simulink library "Atmospheric_lib"  (R2020a)
settings: Solver=VariableStepAuto  StartTime=0.0  StopTime=10.0  RelTol=1e-3
settings Model: Creator=muril  LastModifiedBy=muril

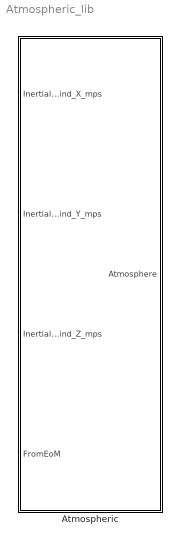
== system Atmospheric_lib ==
  Atmospheric : Subsystem

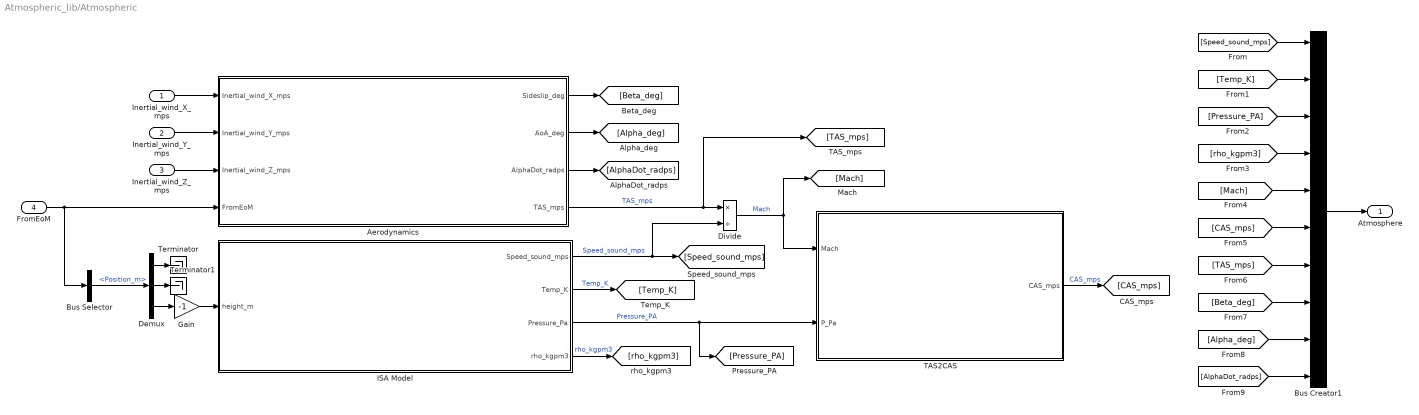
== system Atmospheric_lib/Atmospheric ==
  Inertial_wind_X_mps : Inport
  Inertial_wind_Y_mps : Inport  Port=2
  Inertial_wind_Z_mps : Inport  Port=3
  FromEoM : Inport  Port=4
  Aerodynamics : Subsystem
  Bus Creator1 : BusCreator  Inputs=10
  Bus Selector : BusSelector  OutputSignals=Position_m
  Demux : Demux  Outputs=3
  Divide : Product  Inputs=*/
  Gain : Gain  Gain=-1
  ISA Model : Subsystem
  TAS2CAS : Subsystem
  Terminator : Terminator
  Terminator1 : Terminator
  Atmosphere : Outport
  wires:
  Gain/1 -> ISA Model/1(height_m)
  Bus Selector/1 -> Demux/1  "<Position_m>"
  Demux/2 -> Terminator1/1
  Demux/1 -> Terminator/1
  Demux/3 -> Gain/1
  FromEoM/1 -> Bus Selector/1, Aerodynamics/4(FromEoM)
  Aerodynamics/4(TAS_mps) -> [TAS_mps], Divide/1  "TAS_mps"
  [Speed_sound_mps] -> Bus Creator1/1
  [TAS_mps] -> Bus Creator1/7
  ISA Model/3(Pressure_Pa) -> TAS2CAS/2(P_Pa), [Pressure_PA]  "Pressure_PA"
  ISA Model/4(rho_kgpm3) -> [rho_kgpm3]  "rho_kgpm3"
  ISA Model/1(Speed_sound_mps) -> [Speed_sound_mps], Divide/2  "Speed_sound_mps"
  Aerodynamics/3(AlphaDot_radps) -> [AlphaDot_radps]
  [Pressure_PA] -> Bus Creator1/3
  Divide/1 -> [Mach], TAS2CAS/1(Mach)  "Mach"
  [Alpha_deg] -> Bus Creator1/9
  Inertial_wind_Z_mps/1 -> Aerodynamics/3(Inertial_wind_Z_mps)
  Aerodynamics/1(Sideslip_deg) -> [Beta_deg]
  ISA Model/2(Temp_K) -> [Temp_K]  "Temp_K"
  Aerodynamics/2(AoA_deg) -> [Alpha_deg]
  TAS2CAS/1(CAS_mps) -> [CAS_mps]  "CAS_mps"
  [CAS_mps] -> Bus Creator1/6
  [rho_kgpm3] -> Bus Creator1/4
  Inertial_wind_Y_mps/1 -> Aerodynamics/2(Inertial_wind_Y_mps)
  Inertial_wind_X_mps/1 -> Aerodynamics/1(Inertial_wind_X_mps)
  [AlphaDot_radps] -> Bus Creator1/10
  Bus Creator1/1 -> Atmosphere/1
  [Beta_deg] -> Bus Creator1/8
  [Temp_K] -> Bus Creator1/2
  [Mach] -> Bus Creator1/5

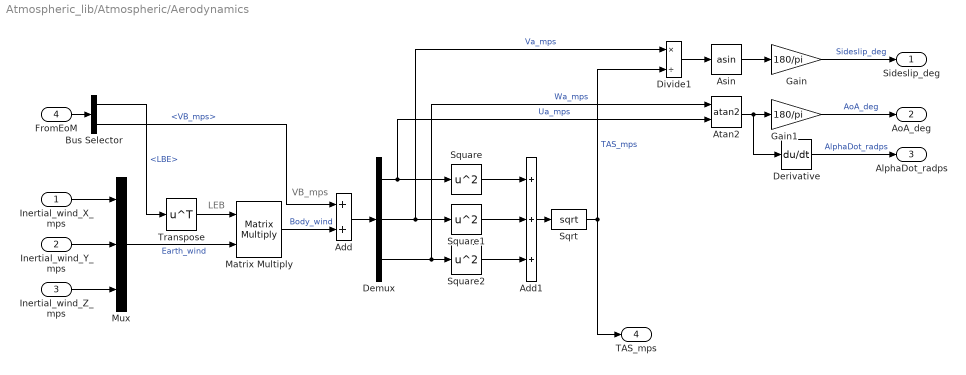
== system Atmospheric_lib/Atmospheric/Aerodynamics ==
  note: LEB
  note: VB_mps
  Inertial_wind_X_mps : Inport
  Inertial_wind_Y_mps : Inport  Port=2
  Inertial_wind_Z_mps : Inport  Port=3
  FromEoM : Inport  Port=4
  Add : Sum
  Add1 : Sum  Inputs=+++
  Asin : Trigonometry  Operator=asin
  Atan2 : Trigonometry  Operator=atan2
  Bus Selector : BusSelector  OutputSignals=LBE,VB_mps
  Demux : Demux  Outputs=3
  Derivative : Derivative
  Divide1 : Product  Inputs=*/
  Gain : Gain  Gain=180/pi
  Gain1 : Gain  Gain=180/pi
  Matrix Multiply : Product  Multiplication=Matrix(*)
  Mux : Mux  Inputs=3
  Sqrt : Sqrt  SaturateOnIntegerOverflow=on
  Square : Math  Operator=square  SaturateOnIntegerOverflow=on
  Square1 : Math  Operator=square  SaturateOnIntegerOverflow=on
  Square2 : Math  Operator=square  SaturateOnIntegerOverflow=on
  Transpose : Math  Operator=transpose  SaturateOnIntegerOverflow=on
  Sideslip_deg : Outport
  AoA_deg : Outport  Port=2
  AlphaDot_radps : Outport  Port=3
  TAS_mps : Outport  Port=4
  wires:
  Derivative/1 -> AlphaDot_radps/1  "AlphaDot_radps"
  Gain/1 -> Sideslip_deg/1  "Sideslip_deg"
  Divide1/1 -> Asin/1
  Inertial_wind_Y_mps/1 -> Mux/2
  Transpose/1 -> Matrix Multiply/1
  Bus Selector/1 -> Transpose/1  "<LBE>"
  Sqrt/1 -> TAS_mps/1, Divide1/2  "TAS_mps"
  Demux/2 -> Square1/1, Divide1/1  "Va_mps"
  Inertial_wind_Z_mps/1 -> Mux/3
  Demux/1 -> Atan2/2, Square/1  "Ua_mps"
  Square/1 -> Add1/1
  Demux/3 -> Square2/1, Atan2/1  "Wa_mps"
  Add1/1 -> Sqrt/1
  Asin/1 -> Gain/1
  Square2/1 -> Add1/3
  Add/1 -> Demux/1
  FromEoM/1 -> Bus Selector/1
  Square1/1 -> Add1/2
  Inertial_wind_X_mps/1 -> Mux/1
  Mux/1 -> Matrix Multiply/2  "Earth_wind"
  Matrix Multiply/1 -> Add/2  "Body_wind"
  Bus Selector/2 -> Add/1  "<VB_mps>"
  Atan2/1 -> Gain1/1, Derivative/1
  Gain1/1 -> AoA_deg/1  "AoA_deg"

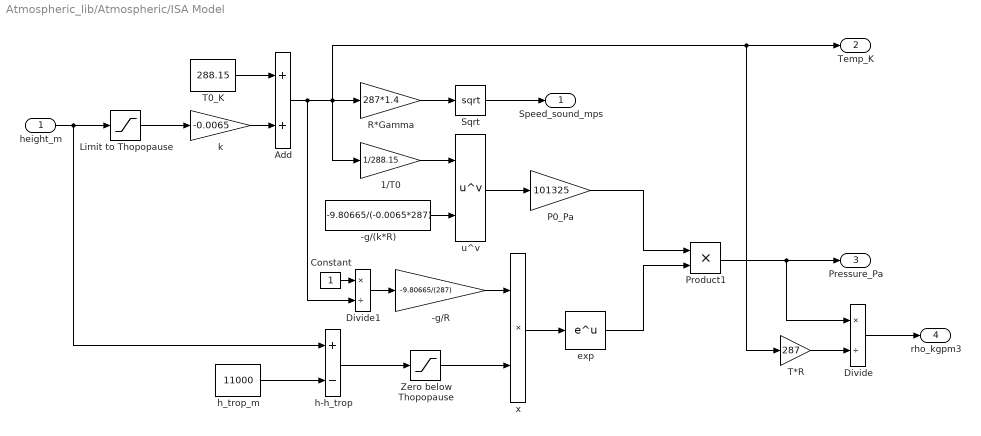
== system Atmospheric_lib/Atmospheric/ISA Model ==
  height_m : Inport
  -g/(k*R) : Constant  Value=-9.80665/(-0.0065*287)
  -g/R : Gain  Gain=-9.80665/(287)
  1/T0 : Gain  Gain=1/288.15
  Add : Sum
  Constant : Constant
  Divide : Product  Inputs=*/
  Divide1 : Product  Inputs=*/
  Limit to Thopopause : Saturate  UpperLimit=11000  LowerLimit=0
  P0_Pa : Gain  Gain=101325
  Product1 : Product
  R*Gamma : Gain  Gain=287*1.4
  Sqrt : Sqrt  SaturateOnIntegerOverflow=on
  T*R : Gain  Gain=287
  T0_K : Constant  Value=288.15
  Zero below Thopopause : Saturate  UpperLimit=inf  LowerLimit=0
  exp : Math  SaturateOnIntegerOverflow=on
  h-h_trop : Sum  Inputs=+-
  h_trop_m : Constant  Value=11000
  k : Gain  Gain=-0.0065
  u^v : Math  Operator=pow  SaturateOnIntegerOverflow=on
  x : Product
  Speed_sound_mps : Outport
  Temp_K : Outport  Port=2
  Pressure_Pa : Outport  Port=3
  rho_kgpm3 : Outport  Port=4
  wires:
  k/1 -> Add/2
  height_m/1 -> Limit to Thopopause/1, h-h_trop/1
  R*Gamma/1 -> Sqrt/1
  Add/1 -> Divide1/2, Temp_K/1, T*R/1, 1/T0/1, R*Gamma/1
  Sqrt/1 -> Speed_sound_mps/1
  T0_K/1 -> Add/1
  Limit to Thopopause/1 -> k/1
  -g/R/1 -> x/1
  -g/(k*R)/1 -> u^v/2
  Zero below Thopopause/1 -> x/2
  Divide/1 -> rho_kgpm3/1
  T*R/1 -> Divide/2
  Divide1/1 -> -g/R/1
  Product1/1 -> Pressure_Pa/1, Divide/1
  1/T0/1 -> u^v/1
  u^v/1 -> P0_Pa/1
  P0_Pa/1 -> Product1/1
  exp/1 -> Product1/2
  h-h_trop/1 -> Zero below Thopopause/1
  x/1 -> exp/1
  h_trop_m/1 -> h-h_trop/2
  Constant/1 -> Divide1/1

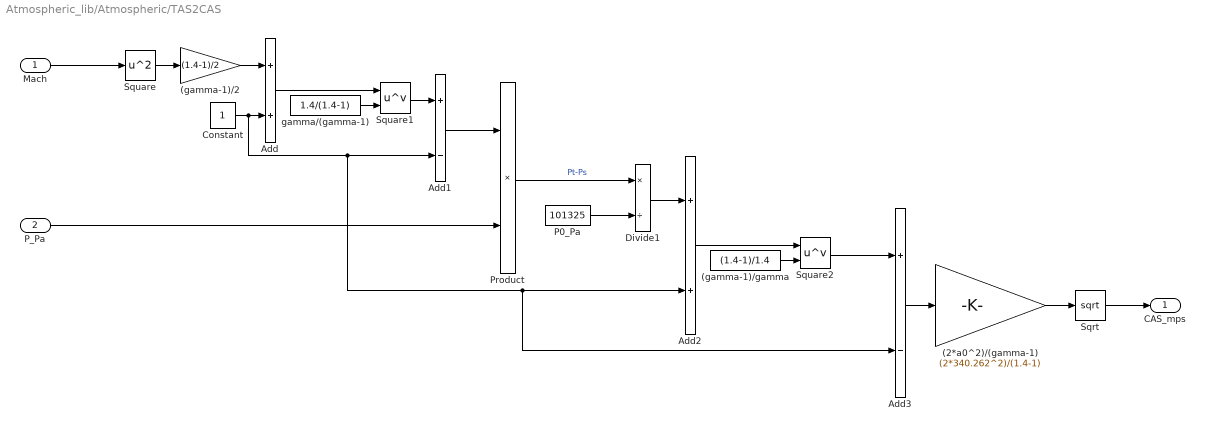
== system Atmospheric_lib/Atmospheric/TAS2CAS ==
  Mach : Inport
  P_Pa : Inport  Port=2
  (2*a0^2)/(gamma-1) : Gain  Gain=(2*340.262^2)/(1.4-1)
  (gamma-1)/2 : Gain  Gain=(1.4-1)/2
  (gamma-1)/gamma : Constant  Value=(1.4-1)/1.4
  Add : Sum
  Add1 : Sum  Inputs=+-
  Add2 : Sum
  Add3 : Sum  Inputs=+-
  Constant : Constant
  Divide1 : Product  Inputs=*/
  P0_Pa : Constant  Value=101325
  Product : Product
  Sqrt : Sqrt  SaturateOnIntegerOverflow=on
  Square : Math  Operator=square  SaturateOnIntegerOverflow=on
  Square1 : Math  Operator=pow  SaturateOnIntegerOverflow=on
  Square2 : Math  Operator=pow  SaturateOnIntegerOverflow=on
  gamma/(gamma-1) : Constant  Value=1.4/(1.4-1)
  CAS_mps : Outport
  wires:
  Constant/1 -> Add3/2, Add2/2, Add1/2, Add/2
  gamma/(gamma-1)/1 -> Square1/2
  Add3/1 -> (2*a0^2)/(gamma-1)/1
  P0_Pa/1 -> Divide1/2
  (gamma-1)/2/1 -> Add/1
  Square1/1 -> Add1/1
  Add/1 -> Square1/1
  Square/1 -> (gamma-1)/2/1
  Sqrt/1 -> CAS_mps/1
  (2*a0^2)/(gamma-1)/1 -> Sqrt/1
  (gamma-1)/gamma/1 -> Square2/2
  Add1/1 -> Product/1
  Add2/1 -> Square2/1
  Product/1 -> Divide1/1  "Pt-Ps"
  Divide1/1 -> Add2/1
  Square2/1 -> Add3/1
  P_Pa/1 -> Product/2
  Mach/1 -> Square/1
